simulink model "ROPOD_dynamic_model_sim_Wheel_Input"  (R2016b)
settings: Solver=FixedStepAuto  StartTime=0.0  StopTime=timesim(end)  FixedStep=Ts  MaxStep=1e-3  RelTol=1e-3
values from neighbouring files (symbols this model uses):
  ropod_dynmodel_pv = struct2array(ropod_dynmodel_param)    [set_ropod_configparams_sim.m]
(part 1 of 4)
settings Model: Creator=cesar  LastModifiedBy=cesar

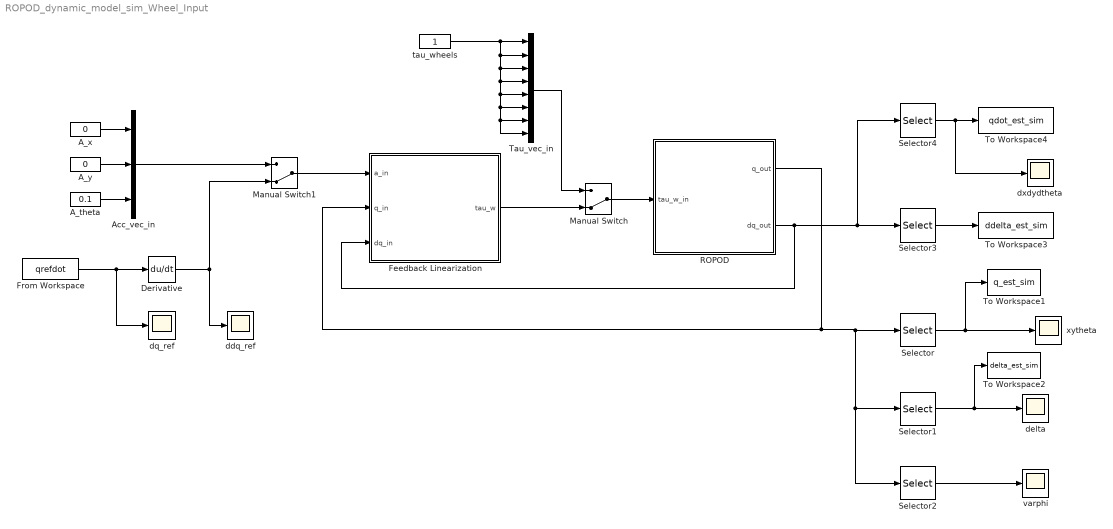
== system ROPOD_dynamic_model_sim_Wheel_Input ==
  A_theta : Constant  Value=0.1
  A_x : Constant  Value=0
  A_y : Constant  Value=0
  Acc_vec_in : Concatenate  NumInputs=3
  Derivative : Derivative
  Feedback Linearization : Subsystem
  From Workspace : FromWorkspace  VariableName=qrefdot  SampleTime=0
  Manual Switch : ManualSwitch  CurrentSetting=0
  Manual Switch1 : ManualSwitch  CurrentSetting=0
  ROPOD : Subsystem
  Selector : Selector  InputPortWidth=15  IndexOptions=Index vector (dialog)  Indices=[1 2 3]  OutputSizes=1
  Selector1 : Selector  InputPortWidth=15  IndexOptions=Index vector (dialog)  Indices=4:7  OutputSizes=1
  Selector2 : Selector  InputPortWidth=15  IndexOptions=Index vector (dialog)  Indices=8:15  OutputSizes=1
  Selector3 : Selector  InputPortWidth=15  IndexOptions=Index vector (dialog)  Indices=4:7  OutputSizes=1
  Selector4 : Selector  InputPortWidth=15  IndexOptions=Index vector (dialog)  Indices=[1 2 3]  OutputSizes=1
  Tau_vec_in : Concatenate  NumInputs=8
  To Workspace1 : ToWorkspace  VariableName=q_est_sim  SaveFormat=Timeseries  SampleTime=-1
  To Workspace2 : ToWorkspace  VariableName=delta_est_sim  SaveFormat=Timeseries  SampleTime=-1
  To Workspace3 : ToWorkspace  VariableName=ddelta_est_sim  SaveFormat=Timeseries  SampleTime=-1
  To Workspace4 : ToWorkspace  VariableName=qdot_est_sim  SaveFormat=Timeseries  SampleTime=-1
  ddq_ref : Scope
  delta : Scope
  dq_ref : Scope
  dxdydtheta : Scope
  tau_wheels : Constant
  varphi : Scope
  xytheta : Scope
  wires:
  Selector/1 -> xytheta/1, To Workspace1/1
  Selector1/1 -> delta/1, To Workspace2/1
  Selector2/1 -> varphi/1
  tau_wheels/1 -> Tau_vec_in/8, Tau_vec_in/7, Tau_vec_in/6, Tau_vec_in/5, Tau_vec_in/4, Tau_vec_in/3, Tau_vec_in/2, Tau_vec_in/1
  A_x/1 -> Acc_vec_in/1
  A_y/1 -> Acc_vec_in/2
  A_theta/1 -> Acc_vec_in/3
  From Workspace/1 -> dq_ref/1, Derivative/1
  Acc_vec_in/1 -> Manual Switch1/1
  Derivative/1 -> ddq_ref/1, Manual Switch1/2
  Selector3/1 -> To Workspace3/1
  Selector4/1 -> dxdydtheta/1, To Workspace4/1
  ROPOD/1(q_out) -> Selector2/1, Selector1/1, Selector/1, Feedback Linearization/2(q_in)
  ROPOD/2(dq_out) -> Feedback Linearization/3(dq_in), Selector4/1, Selector3/1
  Manual Switch/1 -> ROPOD/1(tau_w_in)
  Manual Switch1/1 -> Feedback Linearization/1(a_in)
  Tau_vec_in/1 -> Manual Switch/1
  Feedback Linearization/1(tau_w) -> Manual Switch/2

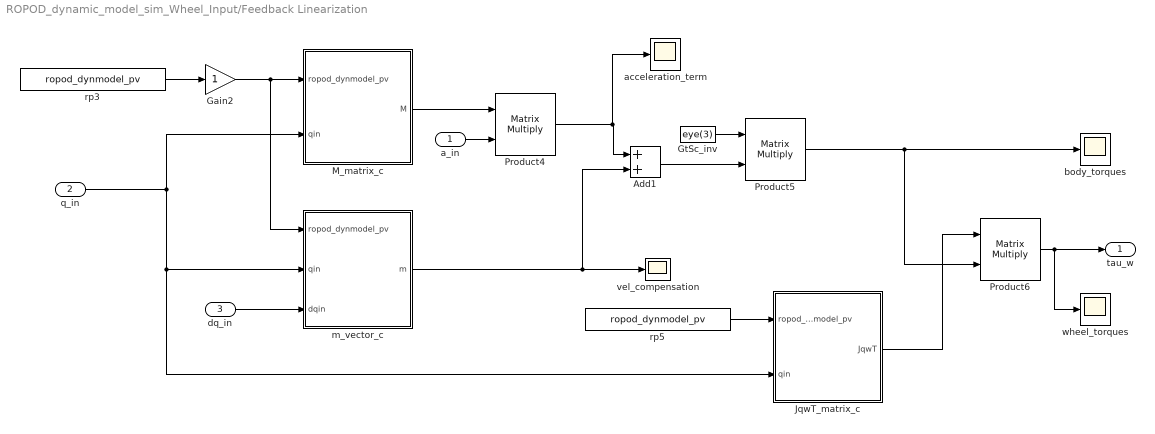
== system ROPOD_dynamic_model_sim_Wheel_Input/Feedback Linearization ==
  a_in : Inport
  q_in : Inport  Port=2
  dq_in : Inport  Port=3
  Add1 : Sum
  Gain2 : Gain
  GtSc_inv : Constant  Value=eye(3)
  JqwT_matrix_c : MATLAB Function  TreatAsAtomicUnit=on
  M_matrix_c : MATLAB Function  TreatAsAtomicUnit=on
  Product4 : Product  Multiplication=Matrix(*)
  Product5 : Product  Multiplication=Matrix(*)
  Product6 : Product  Multiplication=Matrix(*)
  acceleration_term : Scope
  body_torques : Scope
  m_vector_c : MATLAB Function  TreatAsAtomicUnit=on
  rp3 : Constant  Value=ropod_dynmodel_pv  VectorParams1D=off
  rp5 : Constant  Value=ropod_dynmodel_pv  VectorParams1D=off
  vel_compensation : Scope
  wheel_torques : Scope
  tau_w : Outport
  wires:
  q_in/1 -> M_matrix_c/2(qin), JqwT_matrix_c/2(qin), m_vector_c/2(qin)
  dq_in/1 -> m_vector_c/3(dqin)
  rp3/1 -> Gain2/1
  M_matrix_c/1(M) -> Product4/1
  a_in/1 -> Product4/2
  Add1/1 -> Product5/2
  GtSc_inv/1 -> Product5/1
  Product5/1 -> Product6/2, body_torques/1
  Product4/1 -> acceleration_term/1, Add1/1
  rp5/1 -> JqwT_matrix_c/1(ropod_dynmodel_pv)
  Product6/1 -> wheel_torques/1, tau_w/1
  JqwT_matrix_c/1(JqwT) -> Product6/1
  m_vector_c/1(m) -> Add1/2, vel_compensation/1
  Gain2/1 -> m_vector_c/1(ropod_dynmodel_pv), M_matrix_c/1(ropod_dynmodel_pv)

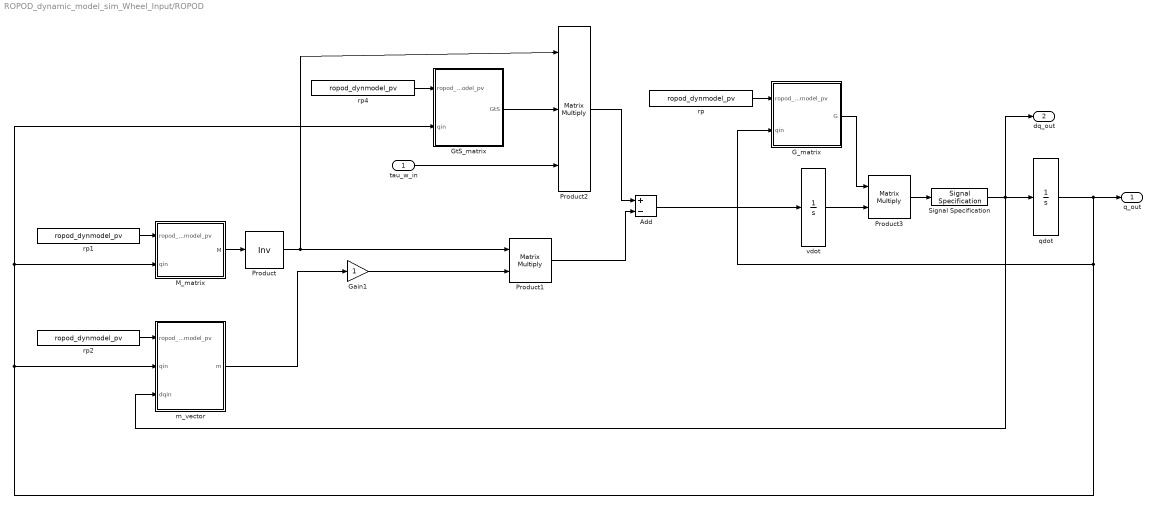
== system ROPOD_dynamic_model_sim_Wheel_Input/ROPOD ==
  tau_w_in : Inport
  Add : Sum  Inputs=+-
  G_matrix : MATLAB Function  TreatAsAtomicUnit=on
  Gain1 : Gain
  GtS_matrix : MATLAB Function  TreatAsAtomicUnit=on
  M_matrix : MATLAB Function  TreatAsAtomicUnit=on
  Product : Product  Inputs=/  Multiplication=Matrix(*)
  Product1 : Product  Multiplication=Matrix(*)
  Product2 : Product  Inputs=3  Multiplication=Matrix(*)
  Product3 : Product  Multiplication=Matrix(*)
  Signal Specification : SignalSpecification  Dimensions=[15 1]
  m_vector : MATLAB Function  TreatAsAtomicUnit=on
  qdot : Integrator  InitialCondition=0*[0 0 0 pi/2 pi/2 pi/2 pi/2 0 0 0 0 0 0 0 0]'
  rp{,1..2,4} (4 alike) : Constant  Value=ropod_dynmodel_pv  VectorParams1D=off
  vdot : Integrator
  q_out : Outport
  dq_out : Outport  Port=2
  wires:
  Signal Specification/1 -> qdot/1, dq_out/1, m_vector/3(dqin)
  Product/1 -> Product2/1, Product1/1
  m_vector/1(m) -> Gain1/1
  Product2/1 -> Add/1
  Product1/1 -> Add/2
  rp/1 -> G_matrix/1(ropod_dynmodel_pv)
  rp1/1 -> M_matrix/1(ropod_dynmodel_pv)
  rp2/1 -> m_vector/1(ropod_dynmodel_pv)
  GtS_matrix/1(GtS) -> Product2/2
  Add/1 -> vdot/1
  Product3/1 -> Signal Specification/1
  G_matrix/1(G) -> Product3/1
  vdot/1 -> Product3/2
  tau_w_in/1 -> Product2/3
  rp4/1 -> GtS_matrix/1(ropod_dynmodel_pv)
  Gain1/1 -> Product1/2
  M_matrix/1(M) -> Product/1
  qdot/1 -> M_matrix/2(qin), GtS_matrix/2(qin), m_vector/2(qin), G_matrix/2(qin), q_out/1

== matlab function ROPOD_dynamic_model_sim_Wheel_Input/ROPOD/M_matrix ==
  data: ropod_dynmodel_pv input; M output; qin input
function M   = M_matrix( ropod_dynmodel_pv, qin)
%ROPOD_JACOBIAN Summary of this function goes here
%   Detailed explanation goes here


r_w     = ropod_dynmodel_pv(1);
s_w     = ropod_dynmodel_pv(2);
d_w     = ropod_dynmodel_pv(3);
l_CW    = ropod_dynmodel_pv(4);

Mr = ropod_dynmodel_pv(5);
Ir = ropod_dynmodel_pv(6);
Mwma = ropod_dynmodel_pv(7);
Iwma = ropod_dynmodel_pv(8);
Mwca = ropod_dynmodel_pv(9);
Iwca = ropod_dynmodel_pv(10);
Mw   = ropod_dynmodel_pv(11);
Iwz  = ropod_dynmodel_pv(12);
Iwp  = ropod_dynmodel_pv(13);


% Map state vector to the corresponfing variables
xc      = qin(1);
yc      = qin(2);
theta   = qin(3);
delta   = qin(4:7);
varphi  = qin(8:15);

delta1 = delta(1);
delta2 = delta(2);
delta3 = delta(3);
delta4 = delta(4);

M = [
[ (4*Iwp*d_w^2 + 8*Iwca*r_w^2 + 8*Iwma*r_w^2 + 16*Iwz*r_w^2 + 16*Iwp*s_w^2 + 4*Mw*d_w^2*r_w^2 + 4*Mr*r_w^2*s_w^2 + 16*Mw*r_w^2*s_w^2 + 10*Mwca*r_w^2*s_w^2 + 8*Mwma*r_w^2*s_w^2 - Iwp*d_w^2*cos(2*delta1 + 2*theta) - Iwp*d_w^2*cos(2*delta2 + 2*theta) - Iwp*d_w^2*cos(2*delta3 + 2*theta) - Iwp*d_w^2*cos(2*delta4 + 2*theta) - 2*Iwca*r_w^2*cos(2*delta1 + 2*theta) - 2*Iwca*r_w^2*cos(2*delta2 + 2*theta) - 2*Iwca*r_w^2*cos(2*delta3 + 2*theta) - 2*Iwca*r_w^2*cos(2*delta4 + 2*theta) - 2*Iwma*r_w^2*cos(2*delta1 + 2*theta) - 2*Iwma*r_w^2*cos(2*delta2 + 2*theta) - 2*Iwma*r_w^2*cos(2*delta3 + 2*theta) - 2*Iwma*r_w^2*cos(2*delta4 + 2*theta) - 4*Iwz*r_w^2*cos(2*delta1 + 2*theta) - 4*Iwz*r_w^2*cos(2*delta2 + 2*theta) - 4*Iwz*r_w^2*cos(2*delta3 + 2*theta) - 4*Iwz*r_w^2*cos(2*delta4 + 2*theta) + 4*Iwp*s_w^2*cos(2*delta1 + 2*theta) + 4*Iwp*s_w^2*cos(2*delta2 + 2*theta) + 4*Iwp*s_w^2*cos(2*delta3 + 2*theta) + 4*Iwp*s_w^2*cos(2*delta4 + 2*theta) - Mw*d_w^2*r_w^2*cos(2*delta1 + 2*theta) - Mw*d_w^2*r_w^2*cos(2*delta2 + 2*theta) - Mw*d_w^2*r_w^2*cos(2*delta3 + 2*theta) - Mw*d_w^2*r_w^2*cos(2*delta4 + 2*theta) + 4*Mw*r_w^2*s_w^2*cos(2*delta1 + 2*theta) + 4*Mw*r_w^2*s_w^2*cos(2*delta2 + 2*theta) + 4*Mw*r_w^2*s_w^2*cos(2*delta3 + 2*theta) + 4*Mw*r_w^2*s_w^2*cos(2*delta4 + 2*theta) + (3*Mwca*r_w^2*s_w^2*cos(2*delta1 + 2*theta))/2 + (3*Mwca*r_w^2*s_w^2*cos(2*delta2 + 2*theta))/2 + (3*Mwca*r_w^2*s_w^2*cos(2*delta3 + 2*theta))/2 + (3*Mwca*r_w^2*s_w^2*cos(2*delta4 + 2*theta))/2 + 2*Mwma*r_w^2*s_w^2*cos(2*delta1 + 2*theta) + 2*Mwma*r_w^2*s_w^2*cos(2*delta2 + 2*theta) + 2*Mwma*r_w^2*s_w^2*cos(2*delta3 + 2*theta) + 2*Mwma*r_w^2*s_w^2*cos(2*delta4 + 2*theta))/(4*r_w^2*s_w^2),                                                                                                                                                                                                                                                                                                                                                                                                                                                                                                                                                                                                                                                                                                                                                                                                                                                                                                                                                                                                                                                                                                                                                                                                                                                                                                                                                                                                                                             -((sin(2*delta1 + 2*theta) + sin(2*delta2 + 2*theta) + sin(2*delta3 + 2*theta) + sin(2*delta4 + 2*theta))*(Iwp*d_w^2 + 2*Iwca*r_w^2 + 2*Iwma*r_w^2 + 4*Iwz*r_w^2 - 4*Iwp*s_w^2 + Mw*d_w^2*r_w^2 - 4*Mw*r_w^2*s_w^2 - (3*Mwca*r_w^2*s_w^2)/2 - 2*Mwma*r_w^2*s_w^2))/(4*r_w^2*s_w^2),                                                                                                                                                                                                                                                                                                                                                                                                                                                                                                                                                                                                                                                                                                                                                                                                                                                                                                                                                                                                                                                                                                                                                                                                                                                                                                                                                                   (2^(1/2)*l_CW*(cos(2*delta1 + theta + pi/4) - cos(2*delta3 + theta + pi/4) - sin(2*delta2 + theta + pi/4) + sin(2*delta4 + theta + pi/4))*(2*Iwp*d_w^2 + 4*Iwca*r_w^2 + 4*Iwma*r_w^2 + 8*Iwz*r_w^2 - 8*Iwp*s_w^2 + 2*Mw*d_w^2*r_w^2 - 8*Mw*r_w^2*s_w^2 - 3*Mwca*r_w^2*s_w^2 - 4*Mwma*r_w^2*s_w^2))/(8*r_w^2*s_w^2)];
[                                                                                                                                                                                                                                                                                                                                                                                                                                                                                                                                                                                                                                                                                                                                                                                                                                                                                                                                                                                                                                                                                                                                                                                                                                                                                                                                                                                                                                             -((sin(2*delta1 + 2*theta) + sin(2*delta2 + 2*theta) + sin(2*delta3 + 2*theta) + sin(2*delta4 + 2*theta))*(Iwp*d_w^2 + 2*Iwca*r_w^2 + 2*Iwma*r_w^2 + 4*Iwz*r_w^2 - 4*Iwp*s_w^2 + Mw*d_w^2*r_w^2 - 4*Mw*r_w^2*s_w^2 - (3*Mwca*r_w^2*s_w^2)/2 - 2*Mwma*r_w^2*s_w^2))/(4*r_w^2*s_w^2), (4*Iwp*d_w^2 + 8*Iwca*r_w^2 + 8*Iwma*r_w^2 + 16*Iwz*r_w^2 + 16*Iwp*s_w^2 + 4*Mw*d_w^2*r_w^2 + 4*Mr*r_w^2*s_w^2 + 16*Mw*r_w^2*s_w^2 + 10*Mwca*r_w^2*s_w^2 + 8*Mwma*r_w^2*s_w^2 + Iwp*d_w^2*cos(2*delta1 + 2*theta) + Iwp*d_w^2*cos(2*delta2 + 2*theta) + Iwp*d_w^2*cos(2*delta3 + 2*theta) + Iwp*d_w^2*cos(2*delta4 + 2*theta) + 2*Iwca*r_w^2*cos(2*delta1 + 2*theta) + 2*Iwca*r_w^2*cos(2*delta2 + 2*theta) + 2*Iwca*r_w^2*cos(2*delta3 + 2*theta) + 2*Iwca*r_w^2*cos(2*delta4 + 2*theta) + 2*Iwma*r_w^2*cos(2*delta1 + 2*theta) + 2*Iwma*r_w^2*cos(2*delta2 + 2*theta) + 2*Iwma*r_w^2*cos(2*delta3 + 2*theta) + 2*Iwma*r_w^2*cos(2*delta4 + 2*theta) + 4*Iwz*r_w^2*cos(2*delta1 + 2*theta) + 4*Iwz*r_w^2*cos(2*delta2 + 2*theta) + 4*Iwz*r_w^2*cos(2*delta3 + 2*theta) + 4*Iwz*r_w^2*cos(2*delta4 + 2*theta) - 4*Iwp*s_w^2*cos(2*delta1 + 2*theta) - 4*Iwp*s_w^2*cos(2*delta2 + 2*theta) - 4*Iwp*s_w^2*cos(2*delta3 + 2*theta) - 4*Iwp*s_w^2*cos(2*delta4 + 2*theta) + Mw*d_w^2*r_w^2*cos(2*delta1 + 2*theta) + Mw*d_w^2*r_w^2*cos(2*delta2 + 2*theta) + Mw*d_w^2*r_w^2*cos(2*delta3 + 2*theta) + Mw*d_w^2*r_w^2*cos(2*delta4 + 2*theta) - 4*Mw*r_w^2*s_w^2*cos(2*delta1 + 2*theta) - 4*Mw*r_w^2*s_w^2*cos(2*delta2 + 2*theta) - 4*Mw*r_w^2*s_w^2*cos(2*delta3 + 2*theta) - 4*Mw*r_w^2*s_w^2*cos(2*delta4 + 2*theta) - (3*Mwca*r_w^2*s_w^2*cos(2*delta1 + 2*theta))/2 - (3*Mwca*r_w^2*s_w^2*cos(2*delta2 + 2*theta))/2 - (3*Mwca*r_w^2*s_w^2*cos(2*delta3 + 2*theta))/2 - (3*Mwca*r_w^2*s_w^2*cos(2*delta4 + 2*theta))/2 - 2*Mwma*r_w^2*s_w^2*cos(2*delta1 + 2*theta) - 2*Mwma*r_w^2*s_w^2*cos(2*delta2 + 2*theta) - 2*Mwma*r_w^2*s_w^2*cos(2*delta3 + 2*theta) - 2*Mwma*r_w^2*s_w^2*cos(2*delta4 + 2*theta))/(4*r_w^2*s_w^2),                                                                                                                                                                                                                                                                                                                                                                                                                                                                                                                                                                                                                                                                                                                                                                                                                                                                                                                                                                                                                                                                                                                                                                                                                                                                                                                                                                   (2^(1/2)*l_CW*(cos(2*delta2 + theta + pi/4) - cos(2*delta4 + theta + pi/4) + sin(2*delta1 + theta + pi/4) - sin(2*delta3 + theta + pi/4))*(2*Iwp*d_w^2 + 4*Iwca*r_w^2 + 4*Iwma*r_w^2 + 8*Iwz*r_w^2 - 8*Iwp*s_w^2 + 2*Mw*d_w^2*r_w^2 - 8*Mw*r_w^2*s_w^2 - 3*Mwca*r_w^2*s_w^2 - 4*Mwma*r_w^2*s_w^2))/(8*r_w^2*s_w^2)];
[                                                                                                                                                                                                                                                                                                                                                                                                                                                                                                                                                                                                                                                                                                                                                                                                                                                                                                                                                                                                                                                                                                                                                                                                                                                                                                                                                                                                             (2^(1/2)*l_CW*(cos(2*delta1 + theta + pi/4) - cos(2*delta3 + theta + pi/4) - sin(2*delta2 + theta + pi/4) + sin(2*delta4 + theta + pi/4))*(2*Iwp*d_w^2 + 4*Iwca*r_w^2 + 4*Iwma*r_w^2 + 8*Iwz*r_w^2 - 8*Iwp*s_w^2 + 2*Mw*d_w^2*r_w^2 - 8*Mw*r_w^2*s_w^2 - 3*Mwca*r_w^2*s_w^2 - 4*Mwma*r_w^2*s_w^2))/(8*r_w^2*s_w^2),                                                                                                                                                                                                                                                                                                                                                                                                                                                                                                                                                                                                                                                                                                                                                                                                                                                                                                                                                                                                                                                                                                                                                                                                                                                                                                                                                                                                             (2^(1/2)*l_CW*(cos(2*delta2 + theta + pi/4) - cos(2*delta4 + theta + pi/4) + sin(2*delta1 + theta + pi/4) - sin(2*delta3 + theta + pi/4))*(2*Iwp*d_w^2 + 4*Iwca*r_w^2 + 4*Iwma*r_w^2 + 8*Iwz*r_w^2 - 8*Iwp*s_w^2 + 2*Mw*d_w^2*r_w^2 - 8*Mw*r_w^2*s_w^2 - 3*Mwca*r_w^2*s_w^2 - 4*Mwma*r_w^2*s_w^2))/(8*r_w^2*s_w^2), (8*Iwp*d_w^2*l_CW^2 + 16*Iwca*l_CW^2*r_w^2 + 16*Iwma*l_CW^2*r_w^2 + 32*Iwz*l_CW^2*r_w^2 + 32*Iwp*l_CW^2*s_w^2 + 4*Ir*r_w^2*s_w^2 + 8*Mw*d_w^2*l_CW^2*r_w^2 + 32*Mw*l_CW^2*r_w^2*s_w^2 + 20*Mwca*l_CW^2*r_w^2*s_w^2 + 16*Mwma*l_CW^2*r_w^2*s_w^2 + 2*Iwp*d_w^2*l_CW^2*sin(2*delta1) - 2*Iwp*d_w^2*l_CW^2*sin(2*delta2) + 2*Iwp*d_w^2*l_CW^2*sin(2*delta3) - 2*Iwp*d_w^2*l_CW^2*sin(2*delta4) + 4*Iwca*l_CW^2*r_w^2*sin(2*delta1) - 4*Iwca*l_CW^2*r_w^2*sin(2*delta2) + 4*Iwca*l_CW^2*r_w^2*sin(2*delta3) - 4*Iwca*l_CW^2*r_w^2*sin(2*delta4) + 4*Iwma*l_CW^2*r_w^2*sin(2*delta1) - 4*Iwma*l_CW^2*r_w^2*sin(2*delta2) + 4*Iwma*l_CW^2*r_w^2*sin(2*delta3) - 4*Iwma*l_CW^2*r_w^2*sin(2*delta4) + 8*Iwz*l_CW^2*r_w^2*sin(2*delta1) - 8*Iwz*l_CW^2*r_w^2*sin(2*delta2) + 8*Iwz*l_CW^2*r_w^2*sin(2*delta3) - 8*Iwz*l_CW^2*r_w^2*sin(2*delta4) - 8*Iwp*l_CW^2*s_w^2*sin(2*delta1) + 8*Iwp*l_CW^2*s_w^2*sin(2*delta2) - 8*Iwp*l_CW^2*s_w^2*sin(2*delta3) + 8*Iwp*l_CW^2*s_w^2*sin(2*delta4) + 2*Mw*d_w^2*l_CW^2*r_w^2*sin(2*delta1) - 2*Mw*d_w^2*l_CW^2*r_w^2*sin(2*delta2) + 2*Mw*d_w^2*l_CW^2*r_w^2*sin(2*delta3) - 2*Mw*d_w^2*l_CW^2*r_w^2*sin(2*delta4) - 8*Mw*l_CW^2*r_w^2*s_w^2*sin(2*delta1) + 8*Mw*l_CW^2*r_w^2*s_w^2*sin(2*delta2) - 8*Mw*l_CW^2*r_w^2*s_w^2*sin(2*delta3) + 8*Mw*l_CW^2*r_w^2*s_w^2*sin(2*delta4) - 3*Mwca*l_CW^2*r_w^2*s_w^2*sin(2*delta1) + 3*Mwca*l_CW^2*r_w^2*s_w^2*sin(2*delta2) - 3*Mwca*l_CW^2*r_w^2*s_w^2*sin(2*delta3) + 3*Mwca*l_CW^2*r_w^2*s_w^2*sin(2*delta4) - 4*Mwma*l_CW^2*r_w^2*s_w^2*sin(2*delta1) + 4*Mwma*l_CW^2*r_w^2*s_w^2*sin(2*delta2) - 4*Mwma*l_CW^2*r_w^2*s_w^2*sin(2*delta3) + 4*Mwma*l_CW^2*r_w^2*s_w^2*sin(2*delta4))/(4*r_w^2*s_w^2)];
 ];


end

== matlab function ROPOD_dynamic_model_sim_Wheel_Input/ROPOD/G_matrix ==
  data: ropod_dynmodel_pv input; G output; qin input
function G   = G_matrix( ropod_dynmodel_pv, qin)
%ROPOD_JACOBIAN Summary of this function goes here
%   Detailed explanation goes here


r_w     = ropod_dynmodel_pv(1);
s_w     = ropod_dynmodel_pv(2);
d_w     = ropod_dynmodel_pv(3);
l_CW    = ropod_dynmodel_pv(4);

Mr = ropod_dynmodel_pv(5);
Ir = ropod_dynmodel_pv(6);
Mwma = ropod_dynmodel_pv(7);
Iwma = ropod_dynmodel_pv(8);
Mwca = ropod_dynmodel_pv(9);
Iwca = ropod_dynmodel_pv(10);
Mw   = ropod_dynmodel_pv(11);
Iwz  = ropod_dynmodel_pv(12);
Iwp  = ropod_dynmodel_pv(13);

% Map state vector to the corresponfing variables
xc      = qin(1);
yc      = qin(2);
theta   = qin(3);
delta   = qin(4:7);
varphi  = qin(8:15);

delta1 = delta(1);
delta2 = delta(2);
delta3 = delta(3);
delta4 = delta(4);


delta1 = delta(1);
delta2 = delta(2);
delta3 = delta(3);
delta4 = delta(4);

G = [
[                                                             1,                                                             0,                                                                                               0];
[                                                             0,                                                             1,                                                                                               0];
[                                                             0,                                                             0,                                                                                               1];
[                                      -sin(delta1 + theta)/s_w,                                       cos(delta1 + theta)/s_w,                                                   (l_CW*cos(delta1) + l_CW*sin(delta1))/s_w - 1];
[                                      -sin(delta2 + theta)/s_w,                                       cos(delta2 + theta)/s_w,                                                   (l_CW*cos(delta2) - l_CW*sin(delta2))/s_w - 1];
[                                      -sin(delta3 + theta)/s_w,                                       cos(delta3 + theta)/s_w,                                                 - (l_CW*cos(delta3) + l_CW*sin(delta3))/s_w - 1];
[                                      -sin(delta4 + theta)/s_w,                                       cos(delta4 + theta)/s_w,                                                 - (l_CW*cos(delta4) - l_CW*sin(delta4))/s_w - 1];
[ (cos(delta1 + theta) + (d_w*sin(delta1 + theta))/(2*s_w))/r_w, (sin(delta1 + theta) - (d_w*cos(delta1 + theta))/(2*s_w))/r_w, -(l_CW*(d_w*cos(delta1) + 2*s_w*cos(delta1) + d_w*sin(delta1) - 2*s_w*sin(delta1)))/(2*r_w*s_w)];
[ (cos(delta1 + theta) - (d_w*sin(delta1 + theta))/(2*s_w))/r_w, (sin(delta1 + theta) + (d_w*cos(delta1 + theta))/(2*s_w))/r_w,  (l_CW*(d_w*cos(delta1) - 2*s_w*cos(delta1) + d_w*sin(delta1) + 2*s_w*sin(delta1)))/(2*r_w*s_w)];
[ (cos(delta2 + theta) + (d_w*sin(delta2 + theta))/(2*s_w))/r_w, (sin(delta2 + theta) - (d_w*cos(delta2 + theta))/(2*s_w))/r_w,  (l_CW*(2*s_w*cos(delta2) - d_w*cos(delta2) + d_w*sin(delta2) + 2*s_w*sin(delta2)))/(2*r_w*s_w)];
[ (cos(delta2 + theta) - (d_w*sin(delta2 + theta))/(2*s_w))/r_w, (sin(delta2 + theta) + (d_w*cos(delta2 + theta))/(2*s_w))/r_w,  (l_CW*(d_w*cos(delta2) + 2*s_w*cos(delta2) - d_w*sin(delta2) + 2*s_w*sin(delta2)))/(2*r_w*s_w)];
[ (cos(delta3 + theta) + (d_w*sin(delta3 + theta))/(2*s_w))/r_w, (sin(delta3 + theta) - (d_w*cos(delta3 + theta))/(2*s_w))/r_w,  (l_CW*(d_w*cos(delta3) + 2*s_w*cos(delta3) + d_w*sin(delta3) - 2*s_w*sin(delta3)))/(2*r_w*s_w)];
[ (cos(delta3 + theta) - (d_w*sin(delta3 + theta))/(2*s_w))/r_w, (sin(delta3 + theta) + (d_w*cos(delta3 + theta))/(2*s_w))/r_w, -(l_CW*(d_w*cos(delta3) - 2*s_w*cos(delta3) + d_w*sin(delta3) + 2*s_w*sin(delta3)))/(2*r_w*s_w)];
[ (cos(delta4 + theta) + (d_w*sin(delta4 + theta))/(2*s_w))/r_w, (sin(delta4 + theta) - (d_w*cos(delta4 + theta))/(2*s_w))/r_w, -(l_CW*(2*s_w*cos(delta4) - d_w*cos(delta4) + d_w*sin(delta4) + 2*s_w*sin(delta4)))/(2*r_w*s_w)];
[ (cos(delta4 + theta) - (d_w*sin(delta4 + theta))/(2*s_w))/r_w, (sin(delta4 + theta) + (d_w*cos(delta4 + theta))/(2*s_w))/r_w, -(l_CW*(d_w*cos(delta4) + 2*s_w*cos(delta4) - d_w*sin(delta4) + 2*s_w*sin(delta4)))/(2*r_w*s_w)];
];


end
